simulink model "bai29"  (R2016a)
settings: Solver=VariableStepAuto  StartTime=0.0  StopTime=10.0  RelTol=1e-3
settings Model: Creator=vuduc  LastModifiedBy=vuduc

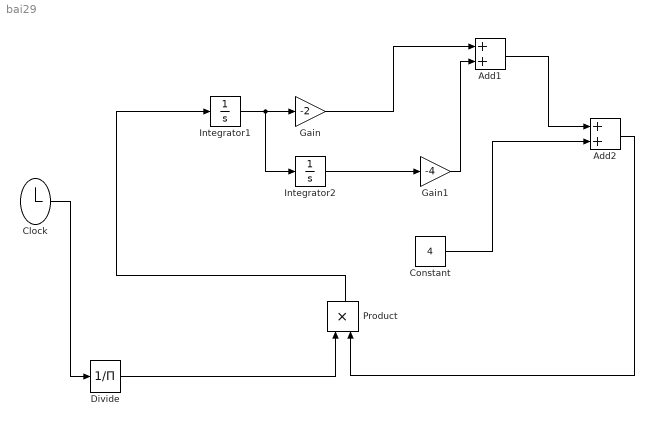
== system bai29 ==
  Add1 : Sum
  Add2 : Sum
  Clock : Clock
  Constant : Constant  Value=4
  Divide : Product  Inputs=/
  Gain : Gain  Gain=-2
  Gain1 : Gain  Gain=-4
  Integrator1 : Integrator  InitialCondition=1
  Integrator2 : Integrator  InitialCondition=1
  Product : Product
  wires:
  Integrator1/1 -> Integrator2/1, Gain/1
  Integrator2/1 -> Gain1/1
  Constant/1 -> Add2/2
  Clock/1 -> Divide/1
  Product/1 -> Integrator1/1
  Gain1/1 -> Add1/2
  Add1/1 -> Add2/1
  Divide/1 -> Product/1
  Add2/1 -> Product/2
  Gain/1 -> Add1/1
